simulink model "model2"  (R2023a)
settings: Solver=VariableStepAuto  StartTime=0.0  StopTime=150  RelTol=1e-3
values from neighbouring files (symbols this model uses):
  data = load(input_data)    [F1.m]    (also in F1Sy.m; F1Vexp2V.m; F1Vexp2V_SexpS.m; F1Vexp2V_SexpS_ssr.m)
  I = A(3)    [F2.m]    (also in F2P1.m; F2P1_ssr.m = input_parameters(3); F2_ssr.m = input_parameters(3); F3.m)
  R = A(2)    [F1.m]    (also in F1Sy.m; F1Vexp2V.m; F1Vexp2V_SexpS.m; F1Vexp2V_SexpS_ssr_all.m = input_parameters(2))
settings Model: Creator=test  LastModifiedBy=test

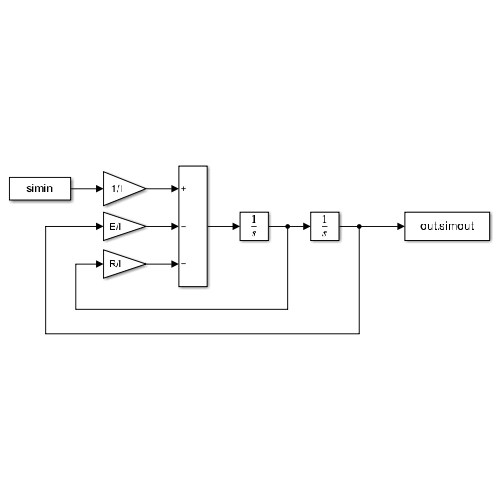
[thumbnail: Simulink's stored preview of the top-level diagram]
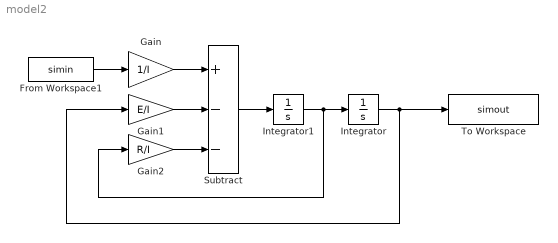
== system model2 ==
  From Workspace1 : FromWorkspace  VariableName=simin
  Gain : Gain  Gain=1/I
  Gain1 : Gain  Gain=E/I
  Gain2 : Gain  Gain=R/I
  Integrator : Integrator  InitialCondition=data(1,3)
  Integrator1 : Integrator  InitialCondition=data(1,2)
  Subtract : Sum  Inputs=+--
  To Workspace : ToWorkspace  VariableName=simout  SaveFormat=Timeseries  SampleTime=0.01
  wires:
  Integrator/1 -> To Workspace/1, Gain1/1
  Gain/1 -> Subtract/1
  From Workspace1/1 -> Gain/1
  Subtract/1 -> Integrator1/1
  Gain1/1 -> Subtract/2
  Integrator1/1 -> Gain2/1, Integrator/1
  Gain2/1 -> Subtract/3
